simulink model "M3b"  (R2021b)
settings: Solver=ode45  StartTime=0.0  StopTime=10.0  MaxStep=0.01  RelTol=1e-3
settings Model: Creator=Student  LastModifiedBy=Student

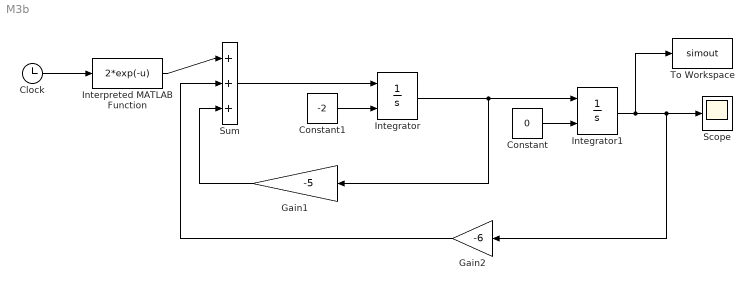
== system M3b ==
  Clock : Clock
  Constant : Constant  Value=0
  Constant1 : Constant  Value=-2
  Gain1 : Gain  Gain=-5
  Gain2 : Gain  Gain=-6
  Integrator : Integrator  InitialConditionSource=external
  Integrator1 : Integrator  InitialConditionSource=external
  Interpreted MATLAB Function : MATLABFcn  MATLABFcn=2*exp(-u)
  Scope : Scope
  Sum : Sum  Inputs=|+++
  To Workspace : ToWorkspace  VariableName=simout  SaveFormat=Timeseries  SampleTime=-1
  wires:
  Gain1/1 -> Sum/3
  Gain2/1 -> Sum/2
  Integrator/1 -> Gain1/1, Integrator1/1
  Constant1/1 -> Integrator/2
  Sum/1 -> Integrator/1
  Constant/1 -> Integrator1/2
  Integrator1/1 -> To Workspace/1, Scope/1, Gain2/1
  Interpreted MATLAB Function/1 -> Sum/1
  Clock/1 -> Interpreted MATLAB Function/1
